simulink model "day5"  (R2017b)
settings: Solver=ode3  StartTime=0.0  StopTime=5000  FixedStep=1  RelTol=1e-3
libraries: SignalEditorBlockLib x1
settings Model: Creator=Admin  LastModifiedBy=Admin

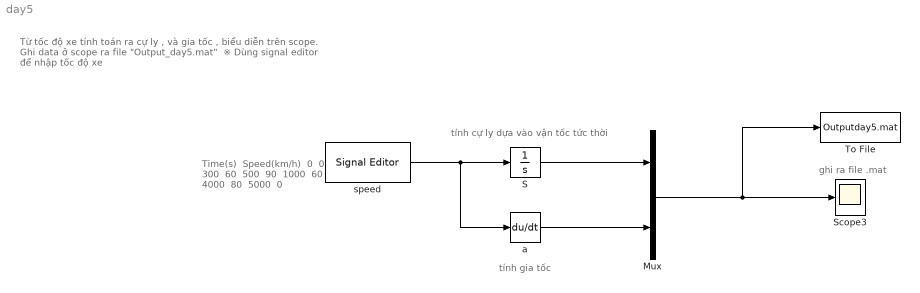
== system day5 ==
  note: tính cự ly dựa vào vận tốc tức thời
  note: Time(s) ​
      | Speed(km/h) ​
      |
      | 0 ​
      | 0 ​
      |
      | 300 ​
      | 60 ​
      |
      | 500 ​
      | 90 ​
      |
      | 1000 ​
      | 60 ​
      |
      | 4000 ​
      | 80 ​
      |
      | 5000 ​
      | 0 ​
  note: Từ tốc độ xe tính toán ra cự ly , và gia tốc , biểu diễn trên scope. ​
      | Ghi data ở scope ra file "Output_day5.mat" ​
      | ※ Dùng signal editor để nhập tốc độ xe ​
      | ​
  note: tính gia tốc
  note: ghi ra file .mat
  Mux : Mux  Inputs=2
  S : Integrator
  Scope3 : Scope
  To File : ToFile  Filename=Outputday5.mat  SaveFormat=Timeseries
  a : Derivative
  "speed " : SignalEditorBlockLib/Signal Editor  FileName=datafile.mat  ActiveScenario=Scenario  ActiveSignal=Signal 1  IsBus=off  OutputBusObjectStr=Bus: BusObject  SampleTime=0  OutputAfterFinalValue=Holding final value  Unit=inherit
  wires:
  "speed "/1 -> a/1, S/1
  S/1 -> Mux/1
  a/1 -> Mux/2
  Mux/1 -> Scope3/1, To File/1
